simulink model "W_client_SOA_demo_codegen"  (R2024b)
settings: Solver=FixedStepAuto  StartTime=0.0  StopTime=10.0  FixedStep=0.2  RelTol=1e-3
settings Model: Tag=EP_AA_WRAPPER_SERVER  Creator=nabilekhoury  LastModifiedBy=nabilekhoury
settings OptimizationCC: DefaultParameterBehavior=Inlined  EnhancedBackFolding=on  PassReuseOutputArgsAs=Individual arguments  ZeroExternalMemoryAtStartup=off  ZeroInternalMemoryAtStartup=off  OptimizeBlockOrder=speed  DifferentSizesBufferReuse=on  OptimizationCustomize=off  EfficientTunableParamExpr=on
settings DebuggingCC: ParameterTunabilityLossMsg=error
settings SFSimCC: MATLABDynamicMemAlloc=off  SimTargetLang=C++
settings RTWCC: Description=Embedded Coder  SystemTargetFile=ert.tlc  GenCodeOnly=on  TemplateMakefile=ert_default_tmf  CustomSourceCode="#include \"SOA_demo_codegen_adapter.h\""  CustomInitializer=sut_initialize();  TargetLang=C++  GPUComputeCapability=3.5
settings CodeAppCC: ForceParamTrailComments=on  IgnoreCustomStorageClasses=off  MaxIdLength=256  OperatorAnnotations=on  SimulinkDataObjDesc=on  SFDataObjDesc=on  CustomSymbolStrGlobalVar=w_$R$N$M  CustomSymbolStrType=w_$N$R$M_T  InsertBlockDesc=on
settings ERTTargetCC: TargetLangStandard=C++11 (ISO)  GenerateSampleERTMain=on  RootIOFormat=Structure reference  ERTCustomFileTemplate=example_file_process.tlc  DynamicArrayContainerType=coder::array

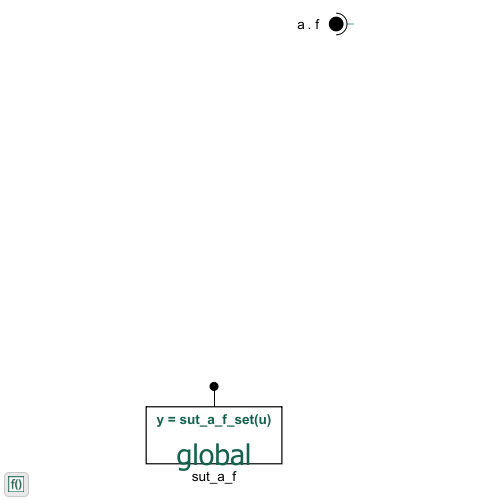
[thumbnail: Simulink's stored preview of the top-level diagram]
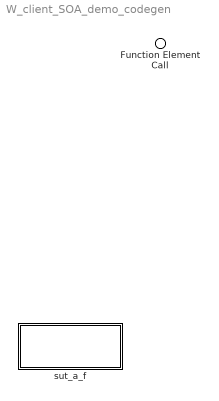
== system W_client_SOA_demo_codegen ==
  Function Element Call : Inport  AllowServiceAccess=on  PortName=a  Element=f
  sut_a_f : Subsystem  TreatAsAtomicUnit=on

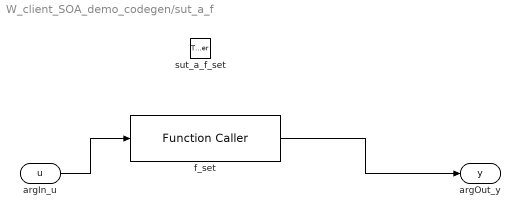
== system W_client_SOA_demo_codegen/sut_a_f ==
  sut_a_f_set : TriggerPort  TriggerType=function-call  IsSimulinkFunction=on  FunctionName=sut_a_f_set  VariantControl=(inherit)
  f_set : FunctionCaller  FunctionPrototype=y = a.f(u)  InputArgumentSpecifications=double(0)  OutputArgumentSpecifications=double(0)
  argIn_u : ArgIn  ArgumentName=u
  argOut_y : ArgOut  ArgumentName=y
  wires:
  argIn_u/1 -> f_set/1
  f_set/1 -> argOut_y/1
